simulink model "small_perturbation_linearized_model_towards"  (R2019b)
settings: Solver=ode4  StartTime=0.0  StopTime=100  FixedStep=1e-3
libraries: dspsrcs4 x1, simulink x1
settings Model: Creator=bitgar  LastModifiedBy=bitgar

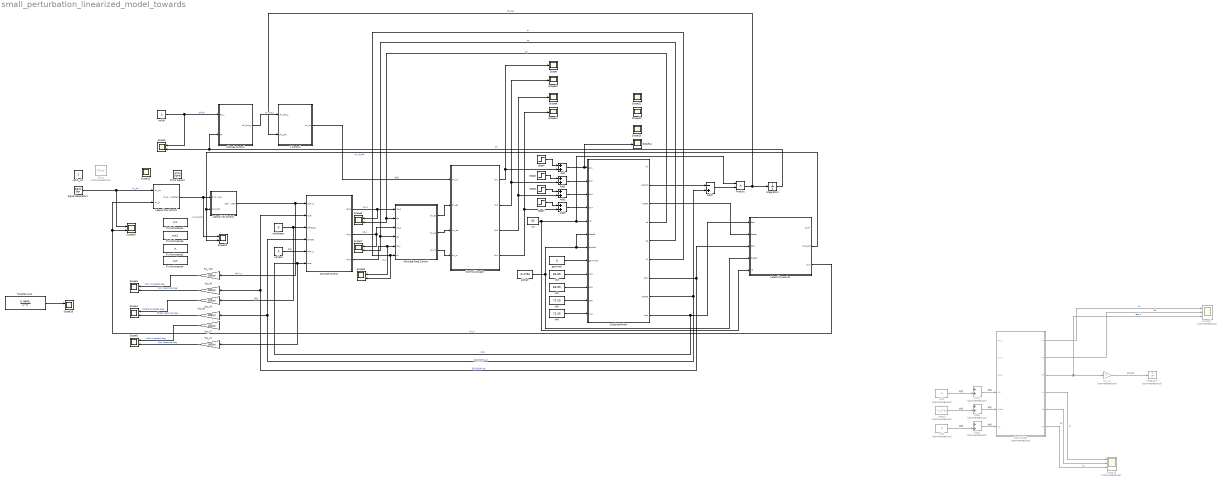
== system small_perturbation_linearized_model_towards ==
  Add{,1..3} (4 alike) : Sum
  Add4 : Sum  Commented=on
  Add5 : Sum  Commented=on
  Add6 : Sum  Commented=on
  Add7 : Sum  Inputs=-+
  Altitude Control : Subsystem
  Attitude Control : Subsystem
  Attitude Rate Control : Subsystem
  BodyToNED : Subsystem  Commented=on
  Chirp : dspsrcs4/Chirp  Commented=on  sweep=Logarithmic  mode=Unidirectional  f0=0.1  f1=150  t1=300  Tsweep=300  phase=1.5*pi  Ts=0.0005  spf=1  datatype=Double  OutputFrames=off
      settings: SourceProductName=DSP System Toolbox
  Chirp Signal1 : simulink/Sources/Chirp Signal  f1=0.1  T=200  f2=200
  ControlAllocator : Subsystem
  Integrator : Integrator  Commented=on
  Integrator1 : Integrator
  Kp_x{1,6..10} (6 alike) : Gain  Gain=180/pi
  Kp_x2 : Gain  Commented=on  Gain=-1
  Lateral Dynamics : Subsystem
  Lateral Pos Control : Subsystem
  Lateral Vel Control : Subsystem
  Product : Product
  QuadrotorPlant : Subsystem
  Scope{,9..15} (8 alike) : Scope
  Scope{1,3..8,16,19..20,22} (11 alike) : Scope  NumInputPorts=2
  Scope17 : Scope  Commented=on  NumInputPorts=3
  Scope18 : Scope  Commented=on  NumInputPorts=3
  Signal Generator1 : SignalGenerator  Frequency=0.1
  Step{4..7} (4 alike) : Step  Time=20  After=0  SampleTime=0
  To Workspace1 : ToWorkspace  VariableName=in1  SampleTime=-1
      settings: Save2DSignal=2-D array (concatenate along first dimension)
  To Workspace2 : ToWorkspace  VariableName=in  SampleTime=-1
      settings: Save2DSignal=2-D array (concatenate along first dimension)
  To Workspace3 : ToWorkspace  VariableName=out1  SampleTime=-1
      settings: Save2DSignal=2-D array (concatenate along first dimension)
  To Workspace4 : ToWorkspace  VariableName=out  SampleTime=-1
      settings: Save2DSignal=2-D array (concatenate along first dimension)
  Transfer Fcn1 : TransferFcn  Numerator=[0.4845]  Denominator=[1 0 0]
  V Control : Subsystem
  V0 : Constant  Value=30
  alpha0 : Constant  Value=-0.4762
  gamma0 : Constant  Value=0
  n10 : Constant  Value=83.85
  n20 : Constant  Value=83.85
  n30 : Constant  Value=72.55
  n40 : Constant  Value=72.55
  phi0 : Constant  Commented=on  Value=0
  psi0 : Constant  Commented=on  Value=0
  ref dh : Constant
  ref dpsi : Constant  Value=0
  ref dtheta : Constant  Value=0
  ref dy_dc : Constant
  theta0 : Constant  Commented=on  Value=-0.4762
  wires:
  Kp_x6/1 -> Scope3/2  "dphi response deg"
  Kp_x8/1 -> Scope4/2  "dtheta response deg"
  QuadrotorPlant/4(dp) -> Scope6/2, Attitude Rate Control/2(dp)  "dp"
  QuadrotorPlant/6(dr) -> Scope8/2, Attitude Rate Control/6(dr)  "dr"
  QuadrotorPlant/7(dphi) -> Lateral Dynamics/3(dphi), Attitude Control/2(dphi), Kp_x6/1  "实际滚转角 rad"
  QuadrotorPlant/8(dtheta) -> Add7/2, Attitude Control/4(dtheta), Kp_x8/1  "实际俯仰角 rad"
  QuadrotorPlant/9(dpsi) -> Lateral Dynamics/1(dpsi), Attitude Control/6(dpsi), Kp_x1/1  "dpsi"
  ref dtheta/1 -> Attitude Control/3(dtheta_c), Kp_x9/1  "期望"
  n10/1 -> QuadrotorPlant/9(n10)
  n20/1 -> QuadrotorPlant/10(n20)
  n30/1 -> QuadrotorPlant/11(n30)
  Kp_x1/1 -> Scope5/2  "dpsi response deg"
  Kp_x7/1 -> Scope5/1  "dpsi expected deg"
  Kp_x9/1 -> Scope4/1  "dtheta expected deg"
  Kp_x10/1 -> Scope3/1  "dphi expected deg"
  ref dh/1 -> Altitude Control/1(dh_c), Scope1/1  "ref dh"
  Kp_x2/1 -> Integrator/1  "dh_dot"
  n40/1 -> QuadrotorPlant/12(n40)
  ControlAllocator/1(dn1) -> Add/2, Scope/1
  ControlAllocator/2(dn2) -> Add1/2, Scope10/1
  ControlAllocator/3(dn3) -> Add2/2, Scope9/1
  ControlAllocator/4(dn4) -> Add3/2, Scope11/1
  QuadrotorPlant/5(dq) -> Attitude Rate Control/4(dq), Scope7/2  "dq"
  Attitude Control/2(dq_c) -> Attitude Rate Control/3(dq_c), Scope7/1  "dq_c"
  Attitude Control/1(dp_c) -> Attitude Rate Control/1(dp_c), Scope6/1  "dp_c"
  Attitude Control/3(dr_c) -> Scope8/1, Attitude Rate Control/5(dr_c)  "dr_c"
  BodyToNED/6(Vd) -> Scope18/3  "vd"
  BodyToNED/3(Pd) -> Kp_x2/1, Scope17/3  "real h"
  BodyToNED/2(Pe) -> Scope17/2  "Pe"
  BodyToNED/5(Ve) -> Scope18/2  "Ve"
  BodyToNED/4(Vn) -> Scope18/1  "Vn"
  BodyToNED/1(Pn) -> Scope17/1  "Pn"
  Add4/1 -> BodyToNED/4(phi)  "期望"
  Add5/1 -> BodyToNED/5(theta)  "期望"
  Add6/1 -> BodyToNED/6(psi)  "期望"
  phi0/1 -> Add4/2  "期望"
  theta0/1 -> Add5/2  "期望"
  psi0/1 -> Add6/2  "期望"
  gamma0/1 -> QuadrotorPlant/8(gamma0)
  alpha0/1 -> QuadrotorPlant/7(alpha0), QuadrotorPlant/6(theta0), Lateral Dynamics/4(theta0)
  V0/1 -> Product/1, QuadrotorPlant/5(V0), Lateral Dynamics/5(V0)
  Step4/1 -> Add/1
  Add/1 -> Scope14/1, QuadrotorPlant/1(dn1)
  Step5/1 -> Add1/1
  Step6/1 -> Add2/1
  Step7/1 -> Add3/1
  Add1/1 -> QuadrotorPlant/2(dn2)
  Add2/1 -> QuadrotorPlant/3(dn3)
  Add3/1 -> QuadrotorPlant/4(dn4)
  Product/1 -> Integrator1/1, V Control/2(dh_dot)  "dh_dot"
  QuadrotorPlant/2(dalpha) -> Add7/1
  Integrator1/1 -> Altitude Control/2(dh), Scope1/2  "dh"
  Altitude Control/1(dh_dot_c) -> V Control/1(dh_dot_c)  "dh_dot_c"
  V Control/1(dn_hc) -> ControlAllocator/1(dn_hc)  "期望"
  Signal Generator1/1 -> Scope16/1, Lateral Pos Control/1(dy_dc)  "dy_dc"
  Lateral Pos Control/1(dy_d_dot_expected) -> Scope20/1, Lateral Vel Control/1(dyd_dot_c)  "dy_d_dotc"
  Lateral Vel Control/1(dphi_c_expected) -> Attitude Control/1(dphi_c), Kp_x10/1  "dphi_c"
  Lateral Dynamics/3(dyd) -> Lateral Pos Control/2(dy_d), Scope16/2  "dy_d"
  QuadrotorPlant/3(dbeta) -> Lateral Dynamics/2(dbeta)
  Add7/1 -> Product/2
  Transfer Fcn1/1 -> Scope19/1
  Attitude Rate Control/1(dn_ec) -> ControlAllocator/2(dn_ec)
  ref dpsi/1 -> Attitude Control/5(dpsi_c)  "期望"
  Attitude Rate Control/2(dn_ac) -> ControlAllocator/3(dn_ac)
  Attitude Rate Control/3(dn_rc) -> ControlAllocator/4(dn_rc)
  Lateral Dynamics/2(dyd_dot) -> Scope20/2, Lateral Vel Control/2(dyd_dot)  "dy_d_dot"

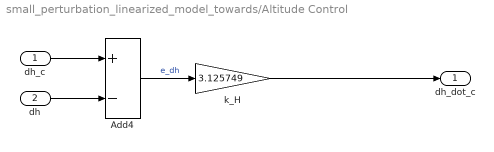
== system small_perturbation_linearized_model_towards/Altitude Control ==
  dh_c : Inport
  dh : Inport  Port=2
  Add4 : Sum  Inputs=+-
  k_H : Gain  Gain=3.125749
  dh_dot_c : Outport
  wires:
  dh_c/1 -> Add4/1
  dh/1 -> Add4/2
  Add4/1 -> k_H/1  "e_dh"
  k_H/1 -> dh_dot_c/1

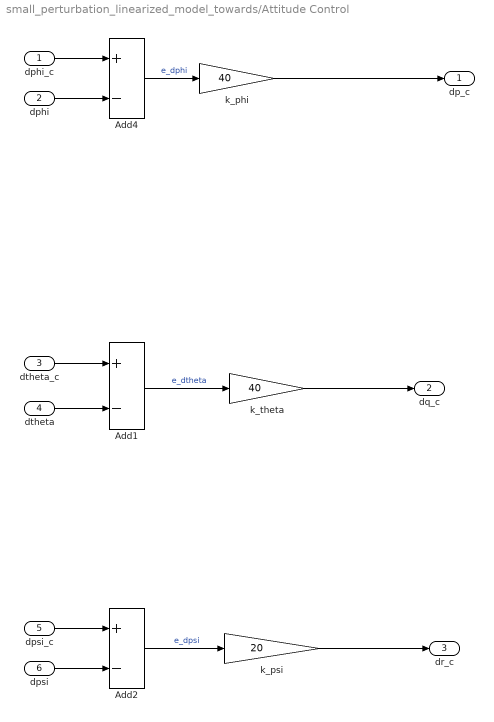
== system small_perturbation_linearized_model_towards/Attitude Control ==
  dphi_c : Inport
  dphi : Inport  Port=2
  dtheta_c : Inport  Port=3
  dtheta : Inport  Port=4
  dpsi_c : Inport  Port=5
  dpsi : Inport  Port=6
  Add1 : Sum  Inputs=+-
  Add2 : Sum  Inputs=+-
  Add4 : Sum  Inputs=+-
  k_phi : Gain  Gain=40
  k_psi : Gain  Gain=20
  k_theta : Gain  Gain=40
  dp_c : Outport
  dq_c : Outport  Port=2
  dr_c : Outport  Port=3
  wires:
  dphi_c/1 -> Add4/1
  dphi/1 -> Add4/2
  dtheta_c/1 -> Add1/1
  dtheta/1 -> Add1/2
  dpsi/1 -> Add2/2
  Add4/1 -> k_phi/1  "e_dphi"
  dpsi_c/1 -> Add2/1
  Add1/1 -> k_theta/1  "e_dtheta"
  Add2/1 -> k_psi/1  "e_dpsi"
  k_phi/1 -> dp_c/1
  k_theta/1 -> dq_c/1
  k_psi/1 -> dr_c/1

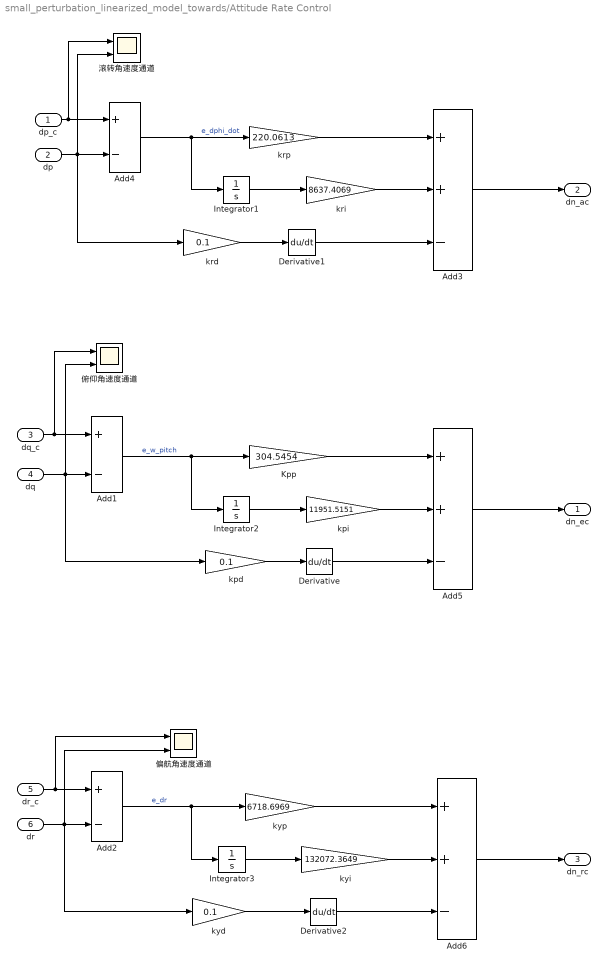
== system small_perturbation_linearized_model_towards/Attitude Rate Control ==
  dp_c : Inport
  dp : Inport  Port=2
  dq_c : Inport  Port=3
  dq : Inport  Port=4
  dr_c : Inport  Port=5
  dr : Inport  Port=6
  Add1 : Sum  Inputs=+-
  Add2 : Sum  Inputs=+-
  Add3 : Sum  Inputs=++-
  Add4 : Sum  Inputs=+-
  Add5 : Sum  Inputs=++-
  Add6 : Sum  Inputs=++-
  Derivative : Derivative
  Derivative1 : Derivative
  Derivative2 : Derivative
  Integrator1 : Integrator
  Integrator2 : Integrator
  Integrator3 : Integrator
  Kpp : Gain  Gain=304.5454
  kpd : Gain  Gain=0.1
  kpi : Gain  Gain=11951.5151
  krd : Gain  Gain=0.1
  kri : Gain  Gain=8637.4069
  krp : Gain  Gain=220.0613
  kyd : Gain  Gain=0.1
  kyi : Gain  Gain=132072.3649
  kyp : Gain  Gain=6718.6969
  俯仰角速度通道 : Scope  NumInputPorts=2
  偏航角速度通道 : Scope  NumInputPorts=2
  滚转角速度通道 : Scope  NumInputPorts=2
  dn_ec : Outport
  dn_ac : Outport  Port=2
  dn_rc : Outport  Port=3
  wires:
  dp_c/1 -> 滚转角速度通道/1, Add4/1
  dp/1 -> krd/1, 滚转角速度通道/2, Add4/2
  dq_c/1 -> 俯仰角速度通道/1, Add1/1
  dq/1 -> kpd/1, 俯仰角速度通道/2, Add1/2
  dr/1 -> 偏航角速度通道/2, kyd/1, Add2/2
  Add4/1 -> Integrator1/1, krp/1  "e_dphi_dot"
  dr_c/1 -> 偏航角速度通道/1, Add2/1
  Add3/1 -> dn_ac/1
  kri/1 -> Add3/2
  krp/1 -> Add3/1
  Integrator1/1 -> kri/1
  Integrator2/1 -> kpi/1
  Kpp/1 -> Add5/1
  kpi/1 -> Add5/2
  Add1/1 -> Integrator2/1, Kpp/1  "e_w_pitch"
  Add5/1 -> dn_ec/1
  Add2/1 -> Integrator3/1, kyp/1  "e_dr"
  Integrator3/1 -> kyi/1
  kyp/1 -> Add6/1
  kyi/1 -> Add6/2
  Add6/1 -> dn_rc/1
  kpd/1 -> Derivative/1
  Derivative/1 -> Add5/3
  krd/1 -> Derivative1/1
  Derivative1/1 -> Add3/3
  kyd/1 -> Derivative2/1
  Derivative2/1 -> Add6/3

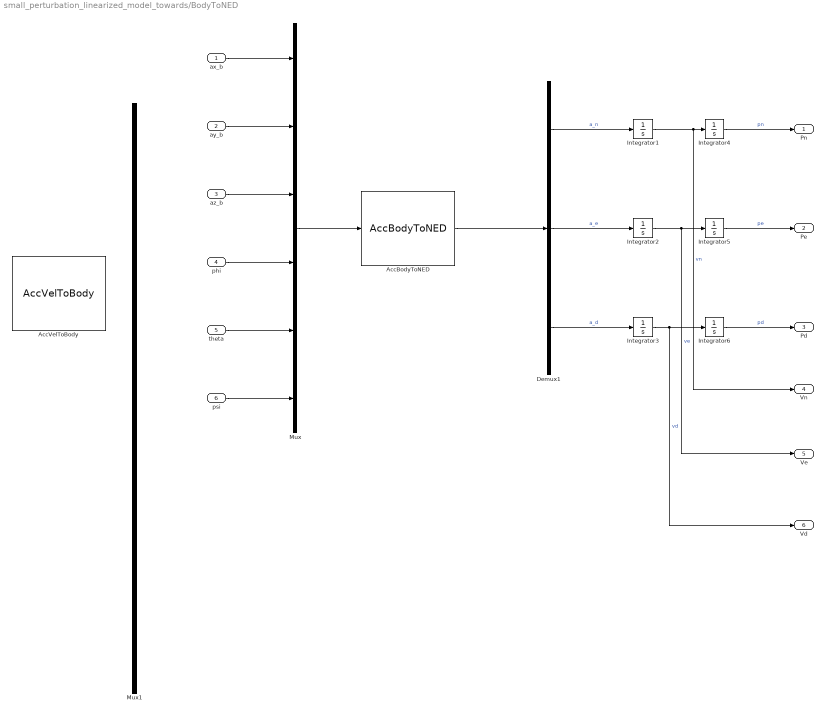
== system small_perturbation_linearized_model_towards/BodyToNED ==
  ax_b : Inport
  ay_b : Inport  Port=2
  az_b : Inport  Port=3
  phi : Inport  Port=4
  theta : Inport  Port=5
  psi : Inport  Port=6
  AccBodyToNED : S-Function  FunctionName=AccBodyToNED  SFunctionDeploymentMode=off  EnableBusSupport=off
  AccVelToBody : S-Function  FunctionName=AccVelToBody  SFunctionDeploymentMode=off  EnableBusSupport=off
  Demux1 : Demux  Outputs=3
  Integrator{1..6} (6 alike) : Integrator
  Mux : Mux  Inputs=6
  Mux1 : Mux  Inputs=6
  Pn : Outport
  Pe : Outport  Port=2
  Pd : Outport  Port=3
  Vn : Outport  Port=4
  Ve : Outport  Port=5
  Vd : Outport  Port=6
  wires:
  az_b/1 -> Mux/3
  psi/1 -> Mux/6
  ax_b/1 -> Mux/1
  ay_b/1 -> Mux/2
  phi/1 -> Mux/4
  theta/1 -> Mux/5
  Demux1/3 -> Integrator3/1  "a_d"
  Demux1/2 -> Integrator2/1  "a_e"
  Demux1/1 -> Integrator1/1  "a_n"
  Integrator1/1 -> Vn/1, Integrator4/1  "vn"
  Integrator2/1 -> Ve/1, Integrator5/1  "ve"
  Integrator3/1 -> Vd/1, Integrator6/1  "vd"
  Integrator4/1 -> Pn/1  "pn"
  Integrator5/1 -> Pe/1  "pe"
  Integrator6/1 -> Pd/1  "pd"
  Mux/1 -> AccBodyToNED/1
  AccBodyToNED/1 -> Demux1/1

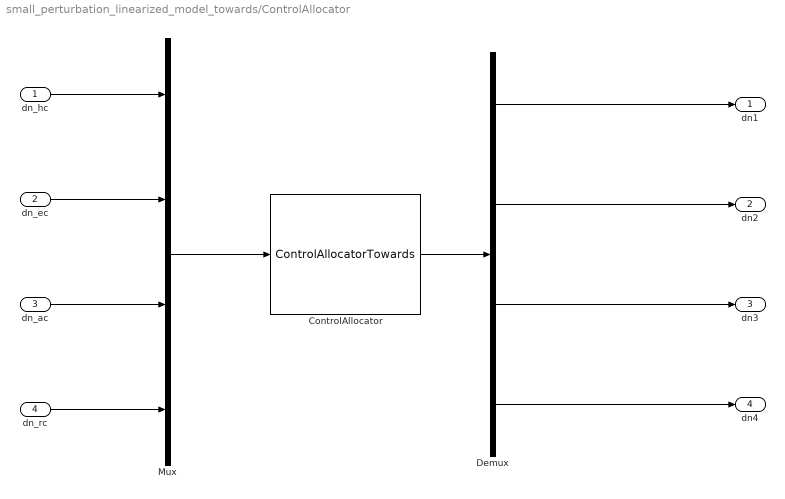
== system small_perturbation_linearized_model_towards/ControlAllocator ==
  dn_hc : Inport
  dn_ec : Inport  Port=2
  dn_ac : Inport  Port=3
  dn_rc : Inport  Port=4
  ControlAllocator : S-Function  FunctionName=ControlAllocatorTowards  Parameters=0.0175 0.0012 0.52 0.7107 -0.1000  SFunctionDeploymentMode=off  EnableBusSupport=off
  Demux : Demux
  Mux : Mux
  dn1 : Outport
  dn2 : Outport  Port=2
  dn3 : Outport  Port=3
  dn4 : Outport  Port=4
  wires:
  Demux/2 -> dn2/1
  Demux/1 -> dn1/1
  Demux/3 -> dn3/1
  Demux/4 -> dn4/1
  Mux/1 -> ControlAllocator/1
  dn_ec/1 -> Mux/2
  dn_ac/1 -> Mux/3
  dn_rc/1 -> Mux/4
  ControlAllocator/1 -> Demux/1
  dn_hc/1 -> Mux/1

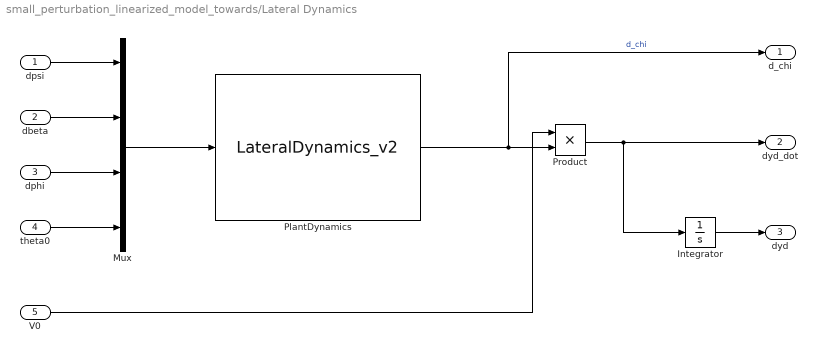
== system small_perturbation_linearized_model_towards/Lateral Dynamics ==
  dpsi : Inport
  dbeta : Inport  Port=2
  dphi : Inport  Port=3
  theta0 : Inport  Port=4
  V0 : Inport  Port=5
  Integrator : Integrator
  Mux : Mux
  PlantDynamics : S-Function  FunctionName=LateralDynamics_v2  Parameters=40.37 9.81 0.52 0.7107 1.375 1.126 -0.1 0.0175 7.7584e-04 0.0012 13.59 9.052 21.238 0.348  SFunctionDeploymentMode=off  EnableBusSupport=off
  Product : Product
  d_chi : Outport
  dyd_dot : Outport  Port=2
  dyd : Outport  Port=3
  wires:
  dpsi/1 -> Mux/1
  dphi/1 -> Mux/3
  theta0/1 -> Mux/4
  Mux/1 -> PlantDynamics/1
  PlantDynamics/1 -> d_chi/1, Product/2  "d_chi"
  Product/1 -> Integrator/1, dyd_dot/1
  Integrator/1 -> dyd/1
  dbeta/1 -> Mux/2
  V0/1 -> Product/1

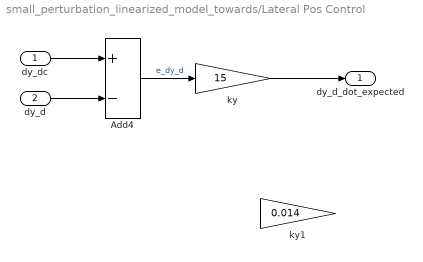
== system small_perturbation_linearized_model_towards/Lateral Pos Control ==
  dy_dc : Inport
  dy_d : Inport  Port=2
  Add4 : Sum  Inputs=+-
  ky : Gain  Gain=15
  ky1 : Gain  Gain=0.014
  dy_d_dot_expected : Outport
  wires:
  dy_dc/1 -> Add4/1
  dy_d/1 -> Add4/2
  Add4/1 -> ky/1  "e_dy_d"
  ky/1 -> dy_d_dot_expected/1

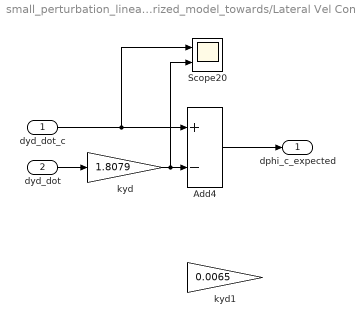
== system small_perturbation_linearized_model_towards/Lateral Vel Control ==
  dyd_dot_c : Inport
  dyd_dot : Inport  Port=2
  Add4 : Sum  Inputs=+-
  Scope20 : Scope  NumInputPorts=2
  kyd : Gain  Gain=1.8079
  kyd1 : Gain  Gain=0.0065
  dphi_c_expected : Outport
  wires:
  dyd_dot_c/1 -> Scope20/1, Add4/1
  dyd_dot/1 -> kyd/1
  Add4/1 -> dphi_c_expected/1
  kyd/1 -> Scope20/2, Add4/2

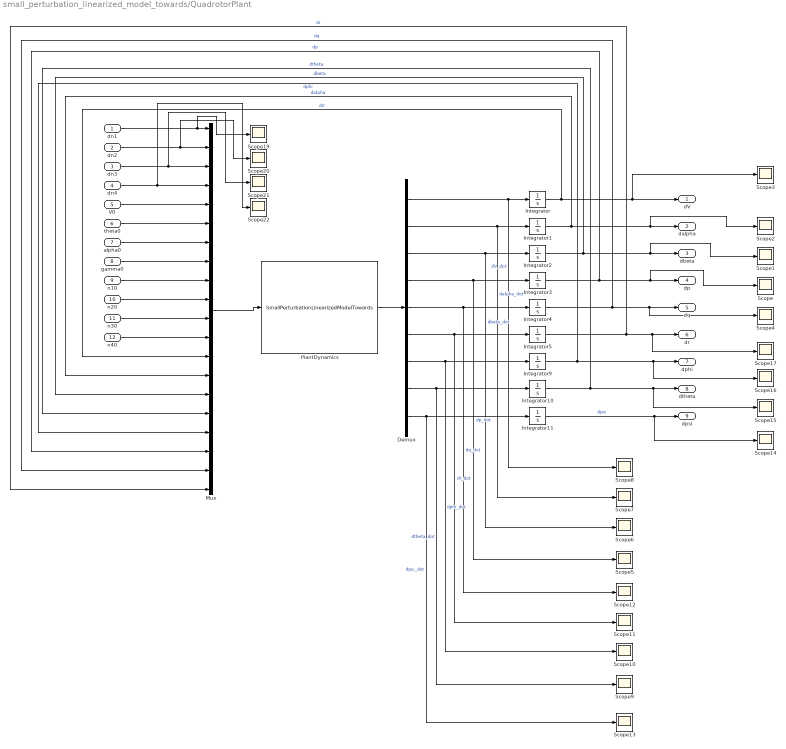
== system small_perturbation_linearized_model_towards/QuadrotorPlant ==
  dn1 : Inport
  dn2 : Inport  Port=2
  dn3 : Inport  Port=3
  dn4 : Inport  Port=4
  V0 : Inport  Port=5
  theta0 : Inport  Port=6
  alpha0 : Inport  Port=7
  gamma0 : Inport  Port=8
  n10 : Inport  Port=9
  n20 : Inport  Port=10
  n30 : Inport  Port=11
  n40 : Inport  Port=12
  Demux : Demux  Outputs=9
  Integrator{,1..5,9..11} (9 alike) : Integrator
  Mux : Mux  Inputs=20
  PlantDynamics : S-Function  FunctionName=SmallPerturbationLinearizedModelTowards  Parameters=40.37 9.81 0.52 0.7107 1.375 1.126 -0.1 1.225 0.309 0.37 0.0175 7.7584e-04 0.0012 13.59 9.052 21.238 0.348  SFunctionDeploymentMode=off  EnableBusSupport=off
  Scope{,1..17,19..22} (22 alike) : Scope
  dV : Outport
  dalpha : Outport  Port=2
  dbeta : Outport  Port=3
  dp : Outport  Port=4
  dq : Outport  Port=5
  dr : Outport  Port=6
  dphi : Outport  Port=7
  dtheta : Outport  Port=8
  dpsi : Outport  Port=9
  wires:
  Demux/4 -> Scope5/1, Integrator3/1  "dp_dot"
  Mux/1 -> PlantDynamics/1
  Demux/3 -> Scope6/1, Integrator2/1  "dbeta_dot"
  dn2/1 -> Scope20/1, Mux/2
  Demux/1 -> Scope8/1, Integrator/1  "dV_dot"
  Demux/5 -> Scope12/1, Integrator4/1  "dq_dot"
  Demux/6 -> Scope11/1, Integrator5/1  "dr_dot"
  Demux/2 -> Scope7/1, Integrator1/1  "dalpha_dot"
  dn4/1 -> Scope22/1, Mux/4
  dn1/1 -> Scope19/1, Mux/1
  dn3/1 -> Scope21/1, Mux/3
  PlantDynamics/1 -> Demux/1
  Integrator9/1 -> Scope16/1, dphi/1, Mux/17  "dphi"
  Integrator10/1 -> Mux/16, Scope15/1, dtheta/1  "dtheta"
  Integrator11/1 -> Scope14/1, dpsi/1  "dpsi"
  Integrator/1 -> Mux/13, Scope3/1, dV/1  "dV"
  Integrator1/1 -> Scope2/1, dalpha/1, Mux/14  "dalpha"
  Integrator2/1 -> Mux/15, Scope1/1, dbeta/1  "dbeta"
  Demux/7 -> Scope10/1, Integrator9/1  "dphi_dot"
  Demux/8 -> Scope9/1, Integrator10/1  "dtheta_dot"
  Demux/9 -> Scope13/1, Integrator11/1  "dpsi_dot"
  Integrator3/1 -> Mux/18, Scope/1, dp/1  "dp"
  Integrator4/1 -> Mux/19, Scope4/1, dq/1  "dq"
  Integrator5/1 -> Mux/20, Scope17/1, dr/1  "dr"
  V0/1 -> Mux/5
  theta0/1 -> Mux/6
  alpha0/1 -> Mux/7
  gamma0/1 -> Mux/8
  n10/1 -> Mux/9
  n20/1 -> Mux/10
  n30/1 -> Mux/11
  n40/1 -> Mux/12

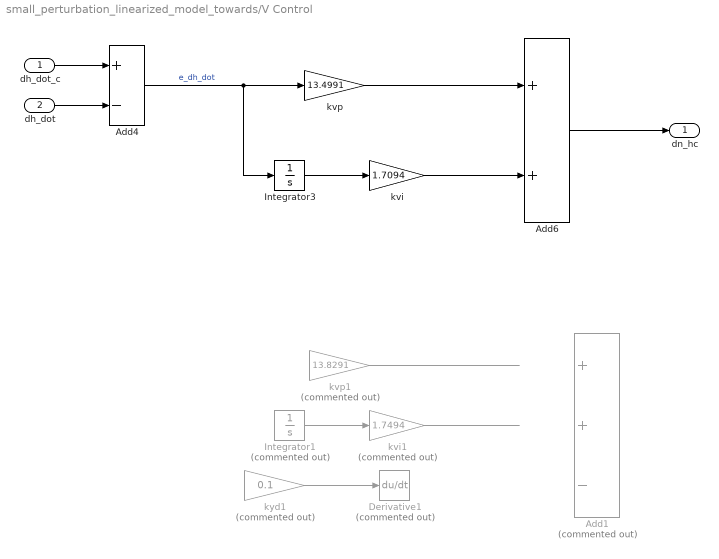
== system small_perturbation_linearized_model_towards/V Control ==
  dh_dot_c : Inport
  dh_dot : Inport  Port=2
  Add1 : Sum  Commented=on  Inputs=++-
  Add4 : Sum  Inputs=+-
  Add6 : Sum
  Derivative1 : Derivative  Commented=on
  Integrator1 : Integrator  Commented=on
  Integrator3 : Integrator
  kvi : Gain  Gain=1.7094
  kvi1 : Gain  Commented=on  Gain=1.7494
  kvp : Gain  Gain=13.4991
  kvp1 : Gain  Commented=on  Gain=13.8291
  kyd1 : Gain  Commented=on  Gain=0.1
  dn_hc : Outport
  wires:
  dh_dot_c/1 -> Add4/1
  dh_dot/1 -> Add4/2
  Add4/1 -> Integrator3/1, kvp/1  "e_dh_dot"
  Add6/1 -> dn_hc/1
  kvi/1 -> Add6/2
  Integrator3/1 -> kvi/1
  kvp/1 -> Add6/1
  kvp1/1 -> ?
  Integrator1/1 -> kvi1/1
  kyd1/1 -> Derivative1/1
  ? -> kvp1/1  "e_dh_dot"
  ? -> Integrator1/1  "e_dh_dot"
  kvi1/1 -> ?
